simulink model "lab2_pid"  (R2022a)
settings: Solver=VariableStepAuto  StartTime=0.0  StopTime=10.0  RelTol=1e-3
settings Model: Creator=bebawy  LastModifiedBy=bebawy

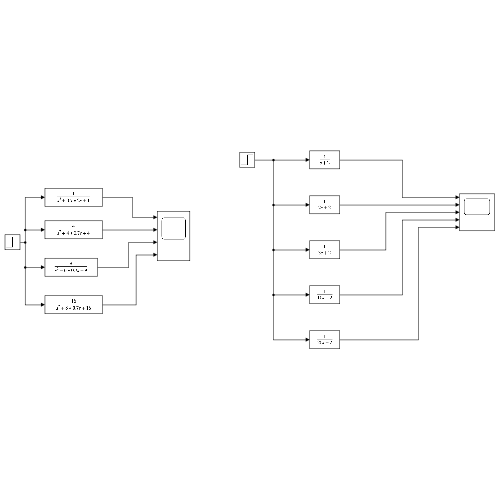
[thumbnail: Simulink's stored preview of the top-level diagram]
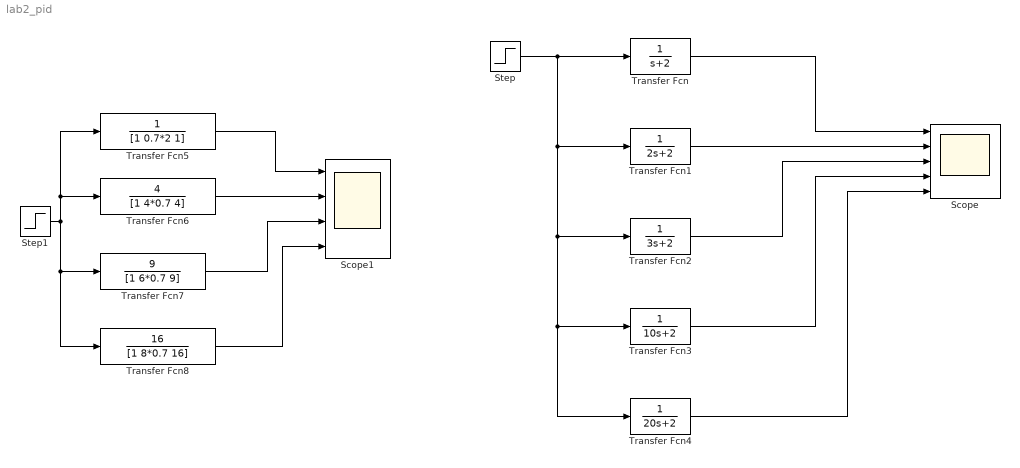
== system lab2_pid ==
  Scope : Scope  NumInputPorts=5
  Scope1 : Scope  NumInputPorts=4
  Step : Step  SampleTime=0
  Step1 : Step  SampleTime=0
  Transfer Fcn : TransferFcn  Denominator=[1 2]
  Transfer Fcn1 : TransferFcn  Denominator=[2 2]
  Transfer Fcn2 : TransferFcn  Denominator=[3 2]
  Transfer Fcn3 : TransferFcn  Denominator=[10 2]
  Transfer Fcn4 : TransferFcn  Denominator=[20 2]
  Transfer Fcn5 : TransferFcn  Denominator=[1 0.7*2 1]
  Transfer Fcn6 : TransferFcn  Numerator=[4]  Denominator=[1 4*0.7 4]
  Transfer Fcn7 : TransferFcn  Numerator=[9]  Denominator=[1 6*0.7 9]
  Transfer Fcn8 : TransferFcn  Numerator=[16]  Denominator=[1 8*0.7 16]
  wires:
  Step/1 -> Transfer Fcn4/1, Transfer Fcn3/1, Transfer Fcn2/1, Transfer Fcn1/1, Transfer Fcn/1
  Transfer Fcn3/1 -> Scope/4
  Transfer Fcn1/1 -> Scope/2
  Transfer Fcn/1 -> Scope/1
  Transfer Fcn2/1 -> Scope/3
  Transfer Fcn4/1 -> Scope/5
  Transfer Fcn5/1 -> Scope1/1
  Step1/1 -> Transfer Fcn5/1, Transfer Fcn6/1, Transfer Fcn8/1, Transfer Fcn7/1
  Transfer Fcn6/1 -> Scope1/2
  Transfer Fcn7/1 -> Scope1/3
  Transfer Fcn8/1 -> Scope1/4
